simulink model "expt_3"  (R2021a)
settings: Solver=VariableStepAuto  StartTime=0.0  StopTime=50  RelTol=1e-3
settings Model: Creator=Kryptic  LastModifiedBy=Kryptic

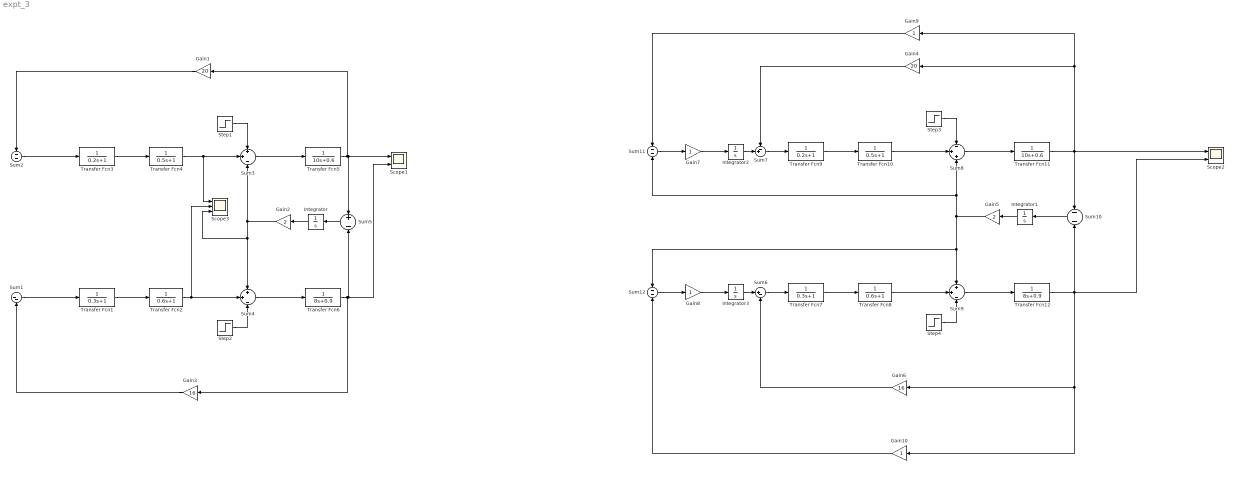
== system expt_3 ==
  Gain1 : Gain  Gain=20
  Gain{7..10} (4 alike) : Gain
  Gain2 : Gain  Gain=2
  Gain3 : Gain  Gain=16
  Gain4 : Gain  Gain=20
  Gain5 : Gain  Gain=2
  Gain6 : Gain  Gain=16
  Integrator{,1..3} (4 alike) : Integrator
  Scope1 : Scope  NumInputPorts=2
  Scope2 : Scope  NumInputPorts=2
  Scope3 : Scope  NumInputPorts=3
  Step1 : Step  Time=0  After=0.1875  SampleTime=0
  Step2 : Step  Time=0  After=0.2  SampleTime=0
  Step3 : Step  Time=0  After=0.1875  SampleTime=0
  Step4 : Step  Time=0  After=0.2  SampleTime=0
  Sum1 : Sum  Inputs=|--
  Sum{2,10..12} (4 alike) : Sum  Inputs=-|-
  Sum3 : Sum  Inputs=+|+|-
  Sum4 : Sum  Inputs=+|+|-
  Sum5 : Sum  Inputs=+|-
  Sum6 : Sum  Inputs=|+-
  Sum7 : Sum  Inputs=-+|
  Sum8 : Sum  Inputs=-|+|+
  Sum9 : Sum  Inputs=+|+|-
  Transfer Fcn1 : TransferFcn  Denominator=[0.3 1]
  Transfer Fcn10 : TransferFcn  Denominator=[0.5 1]
  Transfer Fcn11 : TransferFcn  Denominator=[10 0.6]
  Transfer Fcn12 : TransferFcn  Denominator=[8 0.9]
  Transfer Fcn2 : TransferFcn  Denominator=[0.6 1]
  Transfer Fcn3 : TransferFcn  Denominator=[0.2 1]
  Transfer Fcn4 : TransferFcn  Denominator=[0.5 1]
  Transfer Fcn5 : TransferFcn  Denominator=[10 0.6]
  Transfer Fcn6 : TransferFcn  Denominator=[8 0.9]
  Transfer Fcn7 : TransferFcn  Denominator=[0.3 1]
  Transfer Fcn8 : TransferFcn  Denominator=[0.6 1]
  Transfer Fcn9 : TransferFcn  Denominator=[0.2 1]
  wires:
  Step1/1 -> Sum3/1
  Transfer Fcn3/1 -> Transfer Fcn4/1
  Transfer Fcn5/1 -> Sum5/1, Scope1/1, Gain1/1
  Transfer Fcn4/1 -> Scope3/1, Sum3/2
  Sum2/1 -> Transfer Fcn3/1
  Gain1/1 -> Sum2/1
  Sum3/1 -> Transfer Fcn5/1
  Step2/1 -> Sum4/3
  Transfer Fcn1/1 -> Transfer Fcn2/1
  Transfer Fcn6/1 -> Scope1/2, Sum5/2, Gain3/1
  Transfer Fcn2/1 -> Scope3/2, Sum4/2
  Sum1/1 -> Transfer Fcn1/1
  Gain3/1 -> Sum1/2
  Sum4/1 -> Transfer Fcn6/1
  Integrator/1 -> Gain2/1
  Sum5/1 -> Integrator/1
  Gain2/1 -> Sum3/3, Scope3/3, Sum4/1
  Sum10/1 -> Integrator1/1
  Step4/1 -> Sum9/3
  Sum9/1 -> Transfer Fcn12/1
  Gain6/1 -> Sum6/2
  Sum6/1 -> Transfer Fcn7/1
  Transfer Fcn8/1 -> Sum9/2
  Transfer Fcn12/1 -> Gain10/1, Gain6/1, Scope2/2, Sum10/2
  Transfer Fcn7/1 -> Transfer Fcn8/1
  Sum8/1 -> Transfer Fcn11/1
  Gain4/1 -> Sum7/1
  Transfer Fcn11/1 -> Gain4/1, Gain9/1, Sum10/1, Scope2/1
  Step3/1 -> Sum8/1
  Transfer Fcn9/1 -> Transfer Fcn10/1
  Integrator1/1 -> Gain5/1
  Sum7/1 -> Transfer Fcn9/1
  Transfer Fcn10/1 -> Sum8/2
  Gain5/1 -> Sum11/2, Sum8/3, Sum9/1, Sum12/1
  Gain7/1 -> Integrator2/1
  Gain8/1 -> Integrator3/1
  Integrator2/1 -> Sum7/2
  Sum11/1 -> Gain7/1
  Gain9/1 -> Sum11/1
  Integrator3/1 -> Sum6/1
  Gain10/1 -> Sum12/2
  Sum12/1 -> Gain8/1
